simulink library "NeuroMuscularLibrary"  (R2019a)
settings: Solver=ode45  StartTime=0.0  StopTime=10.0  RelTol=1e-3  EnableMultiTasking=on
undefined symbols (not defined in the file): a2loptHAB, a2loptHAD, a2loptHAMsw, a2loptRFsw, ankle_height, aRefHAB, aRefHAD, aRefHAMsw, aRefRFsw, c, c_jointstop, deltaLegAngleThr, DeltaThRef, eref, Fmax, FmaxGLU, footBallToAnkleDist, footBallToCGDist, footBallToCGDist_y, footBallToHeelDist, footCenterlineToBall, footCenterlineToHeel, footInertia, footLength, footMass, FT, FT_GLU, GainDphiHATGLUst, GainDphiHATHABst, GainDphiHATHADst, GainDphiHATHFLst, GainFGASst, GainFGLUst, GainFHABst, GainFHAMst, GainFSOLst, GainFSOLTAst, GainFVASst, GainLBFSHst, GainLBFSHVASst, GainLGLUsw, GainLHABsw, GainLHADsw, GainLHAMGLUsw, GainLHAMsw, GainLRFHFLsw, GainLTAst, GainLTAsw, GainLVASsw, GainPhiHATGLUst, GainPhiHATHABst, GainPhiHATHADst, GainPhiHATHFLst, GainSGLUcHFLst, GainSGLUHAMst, GainSHABcHABst, GainSHADcHADst, GainSHAMBFSHsw, GainSHAMcHFLst, GainSHAMGASsw ... (+175)
libraries: sm_lib x54, $bdroot x45, nesl_utility x39, simulink x24, simulink_extras x6, vrlib x5, dspsigops x4
(part 1 of 5)
settings Model: Creator=nitisht  LastModifiedBy=Jesper
settings DataIOCC: LimitDataPoints=on  SaveFormat=Array  ReturnWorkspaceOutputs=off
settings OptimizationCC: LifeSpan=inf
settings DebuggingCC: UnderspecifiedInitializationDetection=Classic  MergeDetectMultiDrivingBlocksExec=none  SolverPrmCheckMsg=warning  StateNameClashWarn=warning  SFUnexpectedBacktrackingDiag=warning  SFNoUnconditionalDefaultTransitionDiag=warning  SFExecutionAtInitializationDiag=none  ArithmeticOperatorsInVariantConditions=warning
settings HardwareCC: ProdBitPerLong=64  ProdLargestAtomicFloat=None  ProdIntDivRoundTo=Undefined  ProdEndianess=Unspecified  ProdHWDeviceType=Intel->x86-64
settings ModelReferenceCC: PropagateSignalLabelsOutOfModel=off
settings SFSimCC: SimUseLocalCustomCode=off
settings RTWCC: RTWUseLocalCustomCode=off  RTWCompilerOptimization=on
settings CodeAppCC: StateflowObjectComments=on
settings GRTTargetCC: TargetLangStandard=C89/C90 (ANSI)
settings ConfigComp: CovMetricSettings=dw  CovHtmlReporting=on  CovSaveCumulativeToWorkspaceVar=on  CovSaveSingleToWorkspaceVar=on  CovExternalEMLEnable=off  CovSFcnEnable=off

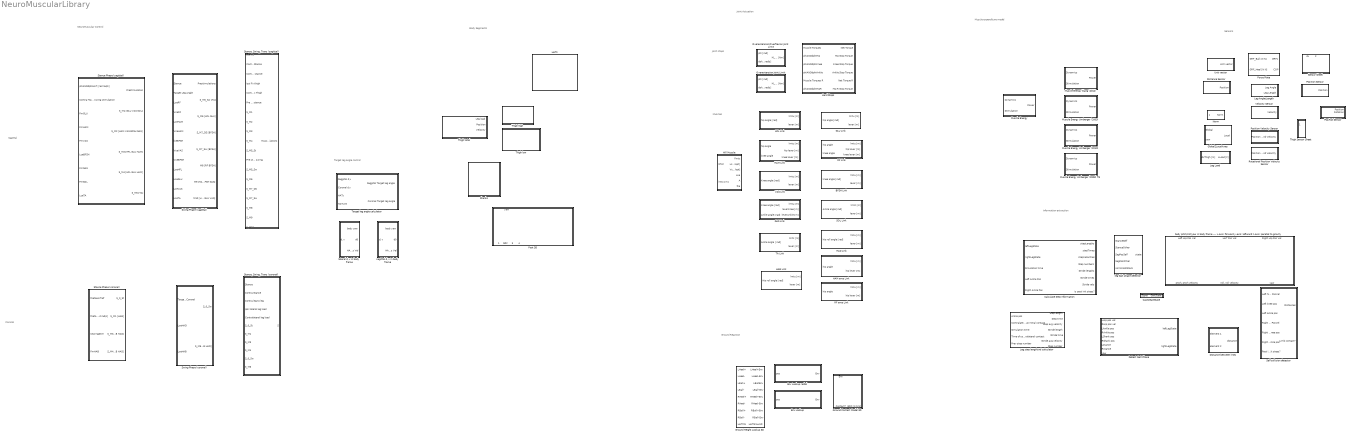
== system NeuroMuscularLibrary ==
  note: Body Segments
  note: Joint Actuation
  note: Sensors
  note: Ground Reaction
  note: NeuroMuscular Control
  note: Sagittal
  note: Coronal
  note: Muscle expenditure
      | model
  note: Joint stops
  note: Muscles
  note: Information extraction
  note: Target leg angle control
  BFSH Link : Subsystem
  Calculate Step information : Subsystem  mask{initiationSteps=innerOptSettings.initiationSteps}
      mask prompts: initiationSteps "Number of initiation steps"
  Cast2GaitState : Subsystem
  Detect Gait Phase : Subsystem
  Distance Sensor : Subsystem
  Distance between lines : Subsystem
  Env Lookup : Subsystem
  Env Lookup radial : Subsystem
  Foot 3D : Subsystem  mask{footMass=footMass, footInertia=footInertia, footSide=Left foot}
      mask prompts: footMass "Foot mass in kg"; footInertia "Foot inertia in kg*m^2"; footSide "Side"
      mask TypeOptions footSide: Left foot | Right foot
  Force Plate : Subsystem  TreatAsAtomicUnit=on
  GAS Link : Subsystem
  GLU Link : Subsystem
  Global2LocalAxes : Subsystem
  Ground Contact Model 3D : Subsystem
  Ground Height Lookup 3D : Subsystem
  HAB Link : Subsystem
  HAD Link : Subsystem
  HAM Link : Subsystem
  HAM amp Link : Subsystem
  HATs : Subsystem
  HFL Link : Subsystem
  Hard Stops : Subsystem
  Hill Muscle : Subsystem  mask(Hill Type Muscle){Fmax=Fmax, lopt=lopt, vmax=vmax, lslack=lslack}
      mask prompts: Fmax "Max Isometric Force [N]"; lopt "Optimal Length [m]"; vmax "Max Contraction Velocity [m/s]"; lslack "Slack Length [m]"
      mask help:
      | Hill Type Muscle Model. This dialog allows you to specify several muscle-specific parameters. The block also requires several parameters to be defined globally in the matlab workspace:
      |
      | Excitation-contraction coupling parameters:
      | preA: preactivation
      | tau:  delay time constant [s]
      |
      | Contractile element (CE) force-length relationship:
      | w: width [lopt]
      | c: remaining force at +/- width
      |
      | CE force-velocity parameters:
      | N: eccentric force enhancement [Fmax]
      | K: shape factor
      |
      | Series elastic element (SE) force-length relationship
      | eref: tendon reference strain [lslack]
  Leg Angle/Length : Subsystem
  Leg Load : Subsystem
  Leg step length/vel calculator : Subsystem
  Muscle Energy : Subsystem  mask{lopt=loptGLU, FT=FT_GLU, Fmax=FmaxGLU, vmax=vmaxGLU}
      mask prompts: lopt "Optimum Length:"; FT "Percent Fast Twitch"; Fmax "Max Iso Force"; vmax "Max Contraction Velocity in m/s"
  Muscle Energy Umberger (2003) : Subsystem  mask{lopt=lopt, FT=FT, Fmax=Fmax, vmax=vmax}
      mask prompts: lopt "Optimum Length:"; FT "Percent Fast Twitch"; Fmax "Max Iso Force"; vmax "Max Contraction Velocity in m/s"
  Muscle Energy Umberger (2003) TG : Subsystem  mask{lopt=loptGLU, FT=FT_GLU, Fmax=FmaxGLU}
      mask prompts: lopt "Optimum Length:"; FT "Percent Fast Twitch"; Fmax "Max Iso Force"
  Muscle Energy Umberger (2010) : Subsystem  mask{lopt=lopt, FT=FT, Fmax=Fmax, vmax=vmax}
      mask prompts: lopt "Optimum Length:"; FT "Percent Fast Twitch"; Fmax "Max Iso Force"; vmax "Max Contraction Velocity in m/s"
  Muscle Energy Wang (2012) : Subsystem  mask{lopt=lopt, FT=FT, Fmax=Fmax}
      mask prompts: lopt "Optimum Length:"; FT "Percent Fast Twitch"; Fmax "Max Iso Force"
  Norm : Subsystem
  Overextension Joint Limit : Subsystem  mask{phiUpLimit=phiKneeUpLimit, ext=1}
      mask prompts: phiUpLimit "Upper Limit [rad]"; ext "Extension values are positive or negative?"
      mask help:
      | This block implements a hard joint limit that will prevent the joint from extending past the specified upper limit.
      |
      | Used for the knee and hip joints.
  Overextension/Overflexion Joint Limit : Subsystem  mask(Overextension/Overflexion Joint Limit){phiUpLimit=0, phiLowLimit=0}
      mask prompts: phiUpLimit "Upper Limit [rad]"; phiLowLimit "Lower Limit [rad]"
      mask help:
      | This block implents a hard joint limit that will prevent the joint from overextending past the specified upper limit and overflexing below the lower limit.
      |
      | Used for the Ankle Joint.
  Pos/Rot Sensor : Subsystem
  Position Sensor : Subsystem
  Position Velocity Sensor : Subsystem
  RF Link : Subsystem
  RF amp Link : Subsystem
  Rotational Position Velocity Sensor : Subsystem
  SOL Link : Subsystem
  Self collision detector : Subsystem  mask{maxDist=innerOptSettings.minLimbDistance}
      mask prompts: maxDist "Minimal distance limbs (m)"
  Sensor Sheet : Subsystem
  Shanks : Subsystem
  Stance Phase (coronal) : Subsystem  TreatAsAtomicUnit=on  mask{PreStimHABst=PreStimHABst, PreStimHADst=PreStimHADst, GainFHABst=GainFHABst, GainPhiHATHABst=GainPhiHATHABst, GainDphiHATHABst=GainDphiHATHABst, GainPhiHATHADst=GainPhiHATHADst, GainDphiHATHADst=GainDphiHATHADst, GainSHABcHABst=GainSHABcHABst, GainSHADcHADst=GainSHADcHADst}
      mask DialogControl Container3 Prompt: Pre-stimulations
      mask DialogControl Container4 Prompt: M1: realize compliant leg
      mask DialogControl Container5 Prompt: M3: balance trunk
      mask DialogControl Container6 Prompt: M4: compensate swing leg
  Stance Phase (sagittal) : Subsystem  TreatAsAtomicUnit=on  mask{PreStimHFLst=PreStimHFLst, PreStimGLUst=PreStimGLUst, PreStimHAMst=PreStimHAMst, PreStimRFst=PreStimRFst, PreStimVASst=PreStimVASst, PreStimBFSHst=PreStimBFSHst, PreStimGASst=PreStimGASst, PreStimSOLst=PreStimSOLst, PreStimTAst=PreStimTAst, GainFGLUst=GainFGLUst, GainFVASst=GainFVASst, GainFSOLst=GainFSOLst, GainFHAMst=GainFHAMst, LceOffsetBFSHVASst=LceOffsetBFSHVASst, GainLBFSHVASst=GainLBFSHVASst, LceOffsetBFSHst=LceOffsetBFSHst, GainLBFSHst=GainLBFSHst, GainFGASst=GainFGASst, phiHATref=phiHATref, GainPhiHATHFLst=GainPhiHATHFLst, GainDphiHATHFLst=GainDphiHATHFLst, GainPhiHATGLUst=GainPhiHATGLUst, GainDphiHATGLUst=GainDphiHATGLUst, GainSGLUHAMst=GainSGLUHAMst, GainSGLUcHFLst=GainSGLUcHFLst, GainSHAMcHFLst=GainSHAMcHFLst, GainSHFLcGLUst=GainSHFLcGLUst, GainSRFcGLUst=GainSRFcGLUst, LceOffsetTAst=LceOffsetTAst, GainLTAst=GainLTAst, GainFSOLTAst=GainFSOLTAst}
      mask DialogControl Container3 Prompt: Pre-stimulations
      mask DialogControl Container4 Prompt: M1: realize compliant leg
      mask DialogControl Container5 Prompt: M2: prevent knee overextension
      mask DialogControl Container6 Prompt: M3: balance trunk
      mask DialogControl Container7 Prompt: M4: compensate swing leg
      mask DialogControl Container8 Prompt: M5: flex ankle
  "Stance, Swing, Trans (coronal)" : Subsystem  TreatAsAtomicUnit=on  mask{transSupst_C=transSupst_C, transsw_C=transsw_C}
  "Stance, Swing, Trans (sagittal)" : Subsystem  mask{transSupst=transSupst, transsw=transsw}
  Swing Phase (coronal) : Subsystem  TreatAsAtomicUnit=on  mask{PreStimHABsw=PreStimHABsw, PreStimHADsw=PreStimHADsw, GainLHABsw=GainLHABsw, GainLHADsw=GainLHADsw}
      mask DialogControl Container2 Prompt: Parameters
      mask DialogControl Container4 Prompt: Pre-stimulations
      mask DialogControl Container5 Prompt: M6: swing hip
  Swing Phase (sagittal) : Subsystem  TreatAsAtomicUnit=on  mask{PreStimHFLsw=PreStimHFLsw, PreStimGLUsw=PreStimGLUsw, PreStimHAMsw=PreStimHAMsw, PreStimRFsw=PreStimRFsw, PreStimVASsw=PreStimVASsw, PreStimBFSHsw=PreStimBFSHsw, PreStimGASsw=PreStimGASsw, PreStimSOLsw=PreStimSOLsw, PreStimTAsw=PreStimTAsw, GainLTAsw=GainLTAsw, LceOffsetTAsw=LceOffsetTAsw, GainLRFHFLsw=GainLRFHFLsw, GainVRFHFLsw=GainVRFHFLsw, GainLHAMGLUsw=GainLHAMGLUsw, GainVHAMGLUsw=GainVHAMGLUsw, GainVRFBFSHsw=GainVRFBFSHsw, GainVVASRFsw=GainVVASRFsw, GainVBFSHsw=GainVBFSHsw, GainLHAMsw=GainLHAMsw, GainSHAMBFSHsw=GainSHAMBFSHsw, GainSHAMGASsw=GainSHAMGASsw, SHAMthresholdsw=SHAMthresholdsw, GainLHFLsw=GainLGLUsw, GainLGLUsw=GainLGLUsw, LceOffsetVASsw=LceOffsetVASsw, GainLVASsw=GainLVASsw, legLengthClr=legLengthClr, deltaLegAngleThr=deltaLegAngleThr}
      mask DialogControl Container4 Prompt: Pre-stimulations
      mask DialogControl Container6 Prompt: M5: swing Ctrl (ankle)
      mask DialogControl Container5 Prompt: M6: swing Ctrl (hip)
      mask DialogControl Container7 Prompt: M7: swing Ctrl (knee_i)
      mask DialogControl Container8 Prompt: swing Ctrl (knee_ii)
      mask DialogControl Container9 Prompt: swing Ctrl (knee_iii)
      mask DialogControl Container10 Prompt: swing Ctrl (stance preparation)
      mask DialogControl Container12 Prompt: Foot placement
  TA Link : Subsystem
  Target leg angle calculator : Subsystem  mask{simbiconLegAngle0=LsimbiconLegAngle0, simbiconGainD=LsimbiconGainD, simbiconGainV=LsimbiconGainV, simbiconLegAngle0_C=LsimbiconLegAngle0_C, simbiconGainD_C=LsimbiconGainD_C, simbiconGainV_C=LsimbiconGainV_C, headingGain=0, headingIntGain=0}
      mask DialogControl Container3 Prompt: Saggital foot placement
      mask DialogControl Container4 Prompt: Coronal foot placement
  Thigh Sensor Sheet : Subsystem
  Thigh high : Subsystem  mask{thighLength=0, thighMass=0, thighInertiaHigh=0, thighKneeToCG=0}
      mask prompts: thighLength "Thigh length (in m)"; thighMass "Thigh mass (in kg)"; thighInertiaHigh "Upper thigh inertia (in kg m^2)"; thighKneeToCG "Distance knee to CG of thigh (in m)"
  Thigh low : Subsystem  mask{thighLength=0, thighMass=0, thighInertiaLow=0, thighKneeToCG=0}
      mask prompts: thighLength "Thigh length (in m)"; thighMass "Thigh mass (in kg)"; thighInertiaLow "Lower thigh inertia (in kg m^2)"; thighKneeToCG "Distance knee to CG of thigh (in m)"
  Thigh total : Subsystem
  Unit vector : Subsystem
  VAS Link : Subsystem
  Velocity Sensor : Subsystem
  body pitch/roll/yaw in body frame --- x-axis: forward y-axis: leftward z-axis: parallel to gravity : Subsystem
  "lateral d, v in body frame" : Subsystem
  leg Gait phase detector : Subsystem
  "sagittal d, v in body frame" : Subsystem

== system NeuroMuscularLibrary/BFSH Link ==
  note: BFSH Attachment
  knee angle [rad] : Inport
  Constant : Constant  Value=lslackBFSH+loptBFSH
  Constant1 : Constant  Value=rBFSH
  Constant2 : Constant  Value=phirefBFSH
  Gain2 : Gain  Gain=rhoBFSH
  Product : Product  RndMeth=Zero
  Sum2 : Sum  Inputs=|-+
  Sum5 : Sum  Inputs=|++
  lmtu [m] : Outport  VectorParamsAs1DForOutWhenUnconnected=on
  lever [m] : Outport  Port=2  VectorParamsAs1DForOutWhenUnconnected=on
  wires:
  Constant1/1 -> Product/2, lever [m]/1
  Constant/1 -> Sum5/1
  Constant2/1 -> Sum2/2
  Sum5/1 -> lmtu [m]/1
  Gain2/1 -> Sum5/2
  Product/1 -> Gain2/1
  knee angle [rad]/1 -> Sum2/1
  Sum2/1 -> Product/1

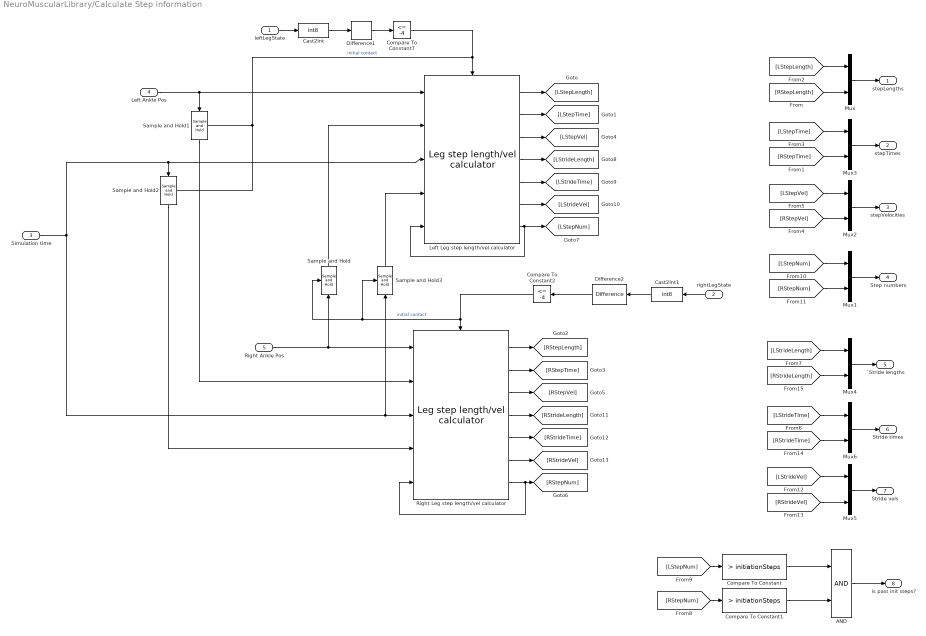
== system NeuroMuscularLibrary/Calculate Step information ==
  leftLegState : Inport
  rightLegState : Inport  Port=2
  Simulation time : Inport  Port=3
  Left Ankle Pos : Inport  Port=4
  "Right Ankle Pos " : Inport  Port=5
  AND : Logic  AllPortsSameDT=off  OutDataTypeStr=boolean
  Cast2Int : DataTypeConversion  OutDataTypeStr=int8
  Cast2Int1 : DataTypeConversion  OutDataTypeStr=int8
  Compare To Constant : simulink/Logic and Bit Operations/Compare To Constant  relop=>  const=initiationSteps  OutDataTypeStr=boolean  ZeroCross=off
  Compare To Constant1 : simulink/Logic and Bit Operations/Compare To Constant  relop=>  const=initiationSteps  OutDataTypeStr=boolean  ZeroCross=off
  Compare To Constant2 : simulink/Logic and Bit Operations/Compare To Constant  relop=<=  const=-4  OutDataTypeStr=boolean
  Compare To Constant7 : simulink/Logic and Bit Operations/Compare To Constant  relop=<=  const=-4  OutDataTypeStr=boolean
  Difference1 : simulink/Discrete/Difference  ICPrevInput=0.0  OutMin=[]  OutMax=[]  OutDataType=fixdt(1, 16)  OutScaling=2^-10  DoSatur=off
  Difference2 : simulink/Discrete/Difference  ICPrevInput=0.0  OutMin=[]  OutMax=[]  OutDataType=fixdt(1, 16)  OutScaling=2^-10  DoSatur=off
  Left Leg step length/vel calculator : $bdroot/Leg step length//vel calculator  SystemSampleTime=-1  Latency=0  AutoFrameSizeCalculation=off
  Mux{,1..6} (7 alike) : Mux  Inputs=2
  Right Leg step length/vel calculator : $bdroot/Leg step length//vel calculator  SystemSampleTime=-1  Latency=0  AutoFrameSizeCalculation=off
  Sample and Hold{,1..3} (4 alike) : dspsigops/Sample and Hold  trig=Rising edge  initCond=0  latchinput=off
  stepLengths : Outport  VectorParamsAs1DForOutWhenUnconnected=on
  stepTimes : Outport  Port=2  VectorParamsAs1DForOutWhenUnconnected=on
  stepVelocities : Outport  Port=3  VectorParamsAs1DForOutWhenUnconnected=on
  Step numbers : Outport  Port=4  VectorParamsAs1DForOutWhenUnconnected=on
  `Stride lengths : Outport  Port=5  VectorParamsAs1DForOutWhenUnconnected=on
  Stride times : Outport  Port=6  VectorParamsAs1DForOutWhenUnconnected=on
  Stride vels : Outport  Port=7  VectorParamsAs1DForOutWhenUnconnected=on
  is past init steps? : Outport  Port=8  VectorParamsAs1DForOutWhenUnconnected=on
  wires:
  Right Leg step length/vel calculator/1 -> [RStepLength]
  Left Leg step length/vel calculator/1 -> [LStepLength]
  Simulation time/1 -> Right Leg step length/vel calculator/3, Sample and Hold3/1, Left Leg step length/vel calculator/3, Sample and Hold2/1
  Compare To Constant7/1 -> Sample and Hold1/Trigger, Sample and Hold2/Trigger, Left Leg step length/vel calculator/Enable  "initial contact"
  Right Leg step length/vel calculator/3 -> [RStepVel]
  Compare To Constant2/1 -> Sample and Hold3/Trigger, Sample and Hold/Trigger, Right Leg step length/vel calculator/Enable  "initial contact"
  Mux2/1 -> stepVelocities/1
  Left Leg step length/vel calculator/3 -> [LStepVel]
  Right Leg step length/vel calculator/2 -> [RStepTime]
  Difference2/1 -> Compare To Constant2/1
  Mux/1 -> stepLengths/1
  Left Leg step length/vel calculator/2 -> [LStepTime]
  Mux3/1 -> stepTimes/1
  leftLegState/1 -> Cast2Int/1
  Compare To Constant1/1 -> AND/2
  Compare To Constant/1 -> AND/1
  AND/1 -> is past init steps?/1
  Left Ankle Pos/1 -> Left Leg step length/vel calculator/1, Sample and Hold1/1
  "Right Ankle Pos "/1 -> Right Leg step length/vel calculator/1, Sample and Hold/1
  Difference1/1 -> Compare To Constant7/1
  rightLegState/1 -> Cast2Int1/1
  [RStepLength] -> Mux/2
  [LStepLength] -> Mux/1
  [LStepTime] -> Mux3/1
  [RStepTime] -> Mux3/2
  [RStepVel] -> Mux2/2
  [LStepVel] -> Mux2/1
  Left Leg step length/vel calculator/7 -> [LStepNum], Left Leg step length/vel calculator/5
  Right Leg step length/vel calculator/7 -> Right Leg step length/vel calculator/5, [RStepNum]
  [LStepNum] -> Compare To Constant/1
  [RStepNum] -> Compare To Constant1/1
  Mux1/1 -> Step numbers/1
  [LStepNum] -> Mux1/1
  [RStepNum] -> Mux1/2
  Left Leg step length/vel calculator/4 -> [LStrideLength]
  Left Leg step length/vel calculator/5 -> [LStrideTime]
  Left Leg step length/vel calculator/6 -> [LStrideVel]
  Right Leg step length/vel calculator/4 -> [RStrideLength]
  Right Leg step length/vel calculator/5 -> [RStrideTime]
  Right Leg step length/vel calculator/6 -> [RStrideVel]
  Sample and Hold/1 -> Left Leg step length/vel calculator/2
  Sample and Hold1/1 -> Right Leg step length/vel calculator/2
  Sample and Hold3/1 -> Left Leg step length/vel calculator/4
  Sample and Hold2/1 -> Right Leg step length/vel calculator/4
  [LStrideVel] -> Mux5/1
  [RStrideLength] -> Mux4/2
  [LStrideTime] -> Mux6/1
  [RStrideTime] -> Mux6/2
  Mux4/1 -> `Stride lengths/1
  [LStrideLength] -> Mux4/1
  Mux6/1 -> Stride times/1
  Mux5/1 -> Stride vels/1
  [RStrideVel] -> Mux5/2
  Cast2Int/1 -> Difference1/1
  Cast2Int1/1 -> Difference2/1

== system NeuroMuscularLibrary/Cast2GaitState ==
  Signal : Inport
  Cast2GaitState : DataTypeConversion  OutDataTypeStr=Enum: GaitState
  Cast2Int : DataTypeConversion  OutDataTypeStr=int8
  GaitState : Outport  OutDataTypeStr=Enum: GaitState  VectorParamsAs1DForOutWhenUnconnected=on
  wires:
  Cast2Int/1 -> Cast2GaitState/1
  Cast2GaitState/1 -> GaitState/1
  Signal/1 -> Cast2Int/1

== system NeuroMuscularLibrary/Detect Gait Phase ==
  LHip pos vel : Inport
  RHip pos vel : Inport  Port=2
  LAnkle pos : Inport  Port=3
  RAnkle pos : Inport  Port=4
  LShank pos : Inport  Port=5
  RShank pos : Inport  Port=6
  Lstance : Inport  Port=7
  Rstance : Inport  Port=8
  yaw : Inport  Port=9
  Add : Sum  Inputs=+-
  Add1 : Sum  Inputs=-+
  Add2 : Sum  Inputs=+-
  Add3 : Sum  Inputs=+-
  Add4 : Sum
  Left leg Gait phase detector : $bdroot/leg Gait phase detector  SystemSampleTime=-1  Latency=0  AutoFrameSizeCalculation=off
  Multiply : Gain  Gain=1/2
  Mux : Mux  Inputs=2
  Mux1 : Mux  Inputs=2
  Norm : Fcn  Expr=sqrt( u(1)^2 + u(2)^2 + u(3)^2 )
  Norm1 : Fcn  Expr=sqrt( u(1)^2 + u(2)^2 + u(3)^2 )
  Right leg Gait phase detector : $bdroot/leg Gait phase detector  SystemSampleTime=-1  Latency=0  AutoFrameSizeCalculation=off
  Selector : Selector  InputPortWidth=3  IndexOptions=Index vector (dialog)  Indices=[1 2]  OutputSizes=1
  Selector1 : Selector  InputPortWidth=3  IndexOptions=Index vector (dialog)  Indices=[1 2]  OutputSizes=1
  Selector4 : Selector  InputPortWidth=6  IndexOptions=Index vector (dialog)  Indices=[1 2 3]  OutputSizes=1
  body frame in transverse plane (xz-plane) : Fcn  Expr=u(1)*cos(u(3)) + u(2)*sin(u(3))
  body frame in transverse plane (xz-plane)1 : Fcn  Expr=u(2)*cos(u(1)) + u(3)*sin(u(1))
  leftLegState : Outport  VectorParamsAs1DForOutWhenUnconnected=on
  rightLegState : Outport  Port=2  VectorParamsAs1DForOutWhenUnconnected=on
  wires:
  LAnkle pos/1 -> Add2/1, Add/1
  RAnkle pos/1 -> Add1/2, Add3/1
  Add/1 -> Selector/1
  Selector/1 -> Mux/1  "(x,y)"
  Add1/1 -> Selector1/1
  Selector1/1 -> Mux1/2  "x,y)"
  LShank pos/1 -> Add2/2
  RShank pos/1 -> Add3/2
  Add3/1 -> Norm1/1
  Add2/1 -> Norm/1
  Add4/1 -> Selector4/1
  Multiply/1 -> Add/2, Add1/1
  LHip pos vel/1 -> Add4/1
  RHip pos vel/1 -> Add4/2
  Selector4/1 -> Multiply/1
  Mux/1 -> body frame in transverse plane (xz-plane)/1
  Mux1/1 -> body frame in transverse plane (xz-plane)1/1
  yaw/1 -> Mux/2, Mux1/1
  body frame in transverse plane (xz-plane)/1 -> [LsagPos]
  body frame in transverse plane (xz-plane)1/1 -> [RsagPos]
  Lstance/1 -> Right leg Gait phase detector/2, Left leg Gait phase detector/1
  Norm1/1 -> [RnormFootShank]
  Norm/1 -> [LnormFootShank]
  [LsagPos] -> Left leg Gait phase detector/3
  [LsagPos] -> Right leg Gait phase detector/4
  [RsagPos] -> Right leg Gait phase detector/3
  [RsagPos] -> Left leg Gait phase detector/4
  [LnormFootShank] -> Left leg Gait phase detector/5
  [RnormFootShank] -> Right leg Gait phase detector/5
  Rstance/1 -> Left leg Gait phase detector/2, Right leg Gait phase detector/1
  Right leg Gait phase detector/1 -> rightLegState/1
  Left leg Gait phase detector/1 -> leftLegState/1

== system NeuroMuscularLibrary/Distance Sensor ==
  PS-Simulink Converter : nesl_utility/PS-Simulink Converter  PhysicalDomain=network_engine_domain  SubClassName=ps_output  LeftPortType=input  RightPortType=output  PseudoPeriodic=off  Frequencies=[]  Unit=m  AffineConversion=off
  Position Sensor : sm_lib/Frames and Transforms/Transform Sensor  MeasurementFrame=World  SenseAngle=off  SenseAxis=off  SenseAngle1=off  SenseAngle2=off  SenseAngle3=off  SenseQ=off  SenseR=off  SenseOmegaX=off  SenseOmegaY=off  SenseOmegaZ=off  SenseOmega1=off  SenseOmega2=off  SenseOmega3=off  SenseQDot=off  SenseRDot=off  SenseAlphaX=off  SenseAlphaY=off  SenseAlphaZ=off  SenseAlpha1=off  SenseAlpha2=off  SenseAlpha3=off  SenseQDDot=off  SenseRDDot=off  SenseX=off  SenseY=off  SenseZ=off  SenseRad=off  SenseAzim=off  SenseDist=on  SenseInc=off  SenseXDot=off  SenseYDot=off  SenseZDot=off  SenseRadDot=off  SenseAzimDot=off  SenseDistDot=off  SenseIncDot=off  SenseXDDot=off  SenseYDDot=off  SenseZDDot=off  SenseRadDDot=off  SenseAzimDDot=off  SenseDistDDot=off  SenseIncDDot=off
  Base : PMIOPort  Side=Left
  Frame : PMIOPort  Port=2  Side=Left
  Position : Outport  VectorParamsAs1DForOutWhenUnconnected=on
  wires:
  PS-Simulink Converter/1 -> Position/1
  connections:
  Base/RConn1 -- Position Sensor/LConn1
  Position Sensor/RConn1 -- Frame/RConn1
  Position Sensor/RConn2 -- PS-Simulink Converter/LConn1

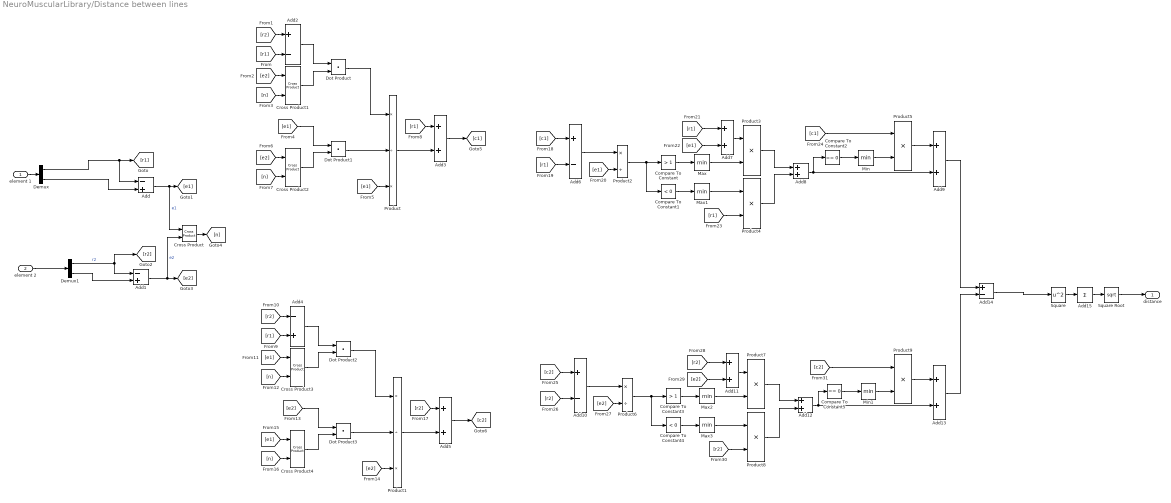
== system NeuroMuscularLibrary/Distance between lines ==
  element 1 : Inport
  element 2 : Inport  Port=2
  Add : Sum  Inputs=-+
  Add1 : Sum  Inputs=-+
  Add{2,6,10,14} (4 alike) : Sum  Inputs=+-
  Add{3,5,7..9,11..13} (8 alike) : Sum
  Add15 : Sum  Inputs=+  CollapseMode=Specified dimension
  Add4 : Sum  Inputs=-+
  Compare To Constant : simulink/Logic and Bit Operations/Compare To Constant  relop=>  const=1  OutDataTypeStr=uint8
  Compare To Constant1 : simulink/Logic and Bit Operations/Compare To Constant  relop=<  const=0  OutDataTypeStr=uint8
  Compare To Constant2 : simulink/Logic and Bit Operations/Compare To Constant  relop===  const=0  OutDataTypeStr=uint8
  Compare To Constant3 : simulink/Logic and Bit Operations/Compare To Constant  relop=>  const=1  OutDataTypeStr=uint8
  Compare To Constant4 : simulink/Logic and Bit Operations/Compare To Constant  relop=<  const=0  OutDataTypeStr=uint8
  Compare To Constant5 : simulink/Logic and Bit Operations/Compare To Constant  relop===  const=0  OutDataTypeStr=uint8
  Cross Product{,1..4} (5 alike) : vrlib/Utilities/Cross Product
  Demux : Demux  Outputs=2
  Demux1 : Demux  Outputs=2
  Dot Product{,1..3} (4 alike) : DotProduct  InputSameDT=on  OutDataTypeStr=Inherit: Inherit via internal rule
  Max{,1..3} (4 alike) : MinMax
  Min : MinMax
  Min1 : MinMax
  Product : Product  Inputs=*/*
  Product1 : Product  Inputs=*/*
  Product2 : Product  Inputs=*/
  Product{3..5,7..9} (6 alike) : Product
  Product6 : Product  Inputs=*/
  Square : Math  Operator=square  SaturateOnIntegerOverflow=on
  Square Root : Sqrt  SaturateOnIntegerOverflow=on
  distance : Outport  VectorParamsAs1DForOutWhenUnconnected=on
  wires:
  Demux/2 -> Add/2
  Demux1/2 -> Add1/2
  Demux1/1 -> [r2], Add1/1  "r2"
  Add/1 -> Cross Product/1, [e1]  "e1"
  Add1/1 -> Cross Product/2, [e2]  "e2"
  Cross Product/1 -> [n]
  [r2] -> Add2/1
  [r1] -> Add2/2
  [e2] -> Cross Product1/1
  [n] -> Cross Product1/2
  Add2/1 -> Dot Product/1
  Cross Product1/1 -> Dot Product/2
  Cross Product2/1 -> Dot Product1/2
  [e1] -> Dot Product1/1
  [n] -> Cross Product2/2
  [e2] -> Cross Product2/1
  Dot Product/1 -> Product/1
  Dot Product1/1 -> Product/2
  [e1] -> Product/3
  [r1] -> Add3/1
  Product/1 -> Add3/2
  Add3/1 -> [c1]
  Add5/1 -> [c2]
  Product1/1 -> Add5/2
  [r2] -> Add5/1
  [e2] -> Product1/3
  Dot Product3/1 -> Product1/2
  Dot Product2/1 -> Product1/1
  [e1] -> Cross Product4/1
  [n] -> Cross Product4/2
  [e2] -> Dot Product3/1
  Cross Product4/1 -> Dot Product3/2
  Cross Product3/1 -> Dot Product2/2
  Add4/1 -> Dot Product2/1
  [n] -> Cross Product3/2
  [e1] -> Cross Product3/1
  [r1] -> Add4/2
  [r2] -> Add4/1
  [r1] -> Add6/2
  [c1] -> Add6/1
  Add6/1 -> Product2/1
  [e1] -> Product2/2
  Product2/1 -> Compare To Constant1/1, Compare To Constant/1
  Compare To Constant/1 -> Max/1
  Compare To Constant1/1 -> Max1/1
  Max/1 -> Product3/2
  Add7/1 -> Product3/1
  [e1] -> Add7/2
  [r1] -> Add7/1
  Max1/1 -> Product4/1
  [r1] -> Product4/2
  Product4/1 -> Add8/2
  Product3/1 -> Add8/1
  [c1] -> Product5/1
  Add8/1 -> Add9/2, Compare To Constant2/1
  Compare To Constant2/1 -> Min/1
  Product5/1 -> Add9/1
  Add9/1 -> Add14/1
  Add12/1 -> Add13/2, Compare To Constant5/1
  Product9/1 -> Add13/1
  [r2] -> Add10/2
  Product8/1 -> Add12/2
  Compare To Constant5/1 -> Min1/1
  [c2] -> Add10/1
  Max2/1 -> Product7/2
  Add13/1 -> Add14/2
  Product7/1 -> Add12/1
  [e2] -> Add11/2
  Add11/1 -> Product7/1
  Compare To Constant3/1 -> Max2/1
  Add10/1 -> Product6/1
  [r2] -> Product8/2
  Product6/1 -> Compare To Constant4/1, Compare To Constant3/1
  Compare To Constant4/1 -> Max3/1
  [r2] -> Add11/1
  Max3/1 -> Product8/1
  [e2] -> Product6/2
  [c2] -> Product9/1
  Add14/1 -> Square/1
  Square Root/1 -> distance/1
  element 1/1 -> Demux/1
  Demux/1 -> Add/1, [r1]
  element 2/1 -> Demux1/1
  Add15/1 -> Square Root/1
  Square/1 -> Add15/1
  Min/1 -> Product5/2
  Min1/1 -> Product9/2

== system NeuroMuscularLibrary/Env Lookup ==
  note: environment lookup
  pos : Inport
  Constant : Constant  Value=0
  Gain : Gain  Gain=-1
  Ground Slope : Interpolation_n-D  NumberOfTableDimensions=1  Table=groundTheta  InterpMethod=Flat
      settings: InputPortMap=u0,u1
  Ground Z : Interpolation_n-D  NumberOfTableDimensions=1  Table=groundZ
      settings: InputPortMap=u0,u1
  Mux : Mux  Inputs=3
  Mux1 : Mux  Inputs=3
  Mux8 : Mux  Inputs=[1 3 3]
  Prelookup : PreLookup  BreakpointsData=groundX  BeginIndexSearchUsingPreviousIndexResult=on  ExtrapMethod=Linear  RndMeth=Simplest
  Selector1 : Selector  InputPortWidth=3  IndexOptions=Index vector (dialog)  Indices=[2]  OutputSizes=1
  Selector2 : Selector  InputPortWidth=3  IndexOptions=Index vector (dialog)  Indices=[1]  OutputSizes=1
  Trigonometric Function1 : Trigonometry
  Trigonometric Function2 : Trigonometry  Operator=cos
  Env : Outport  VectorParamsAs1DForOutWhenUnconnected=on
  wires:
  Constant/1 -> Mux1/2
  Mux1/1 -> Mux8/3  "Normal Vector"
  Selector1/1 -> Mux/2  "y"
  Mux/1 -> Mux8/2  "Reference Point"
  pos/1 -> Selector2/1, Selector1/1
  Prelookup/2 -> Ground Slope/2, Ground Z/2
  Trigonometric Function1/1 -> Gain/1
  Gain/1 -> Mux1/1  "Normal Vector x"
  Ground Slope/1 -> Trigonometric Function2/1, Trigonometric Function1/1
  Prelookup/1 -> Ground Slope/1, Ground Z/1
  Trigonometric Function2/1 -> Mux1/3  "Normal Vector z"
  Selector2/1 -> Prelookup/1, Mux/1  "x"
  Ground Z/1 -> Mux8/1, Mux/3  "Ground Height"
  Mux8/1 -> Env/1

== system NeuroMuscularLibrary/Env Lookup radial ==
  note: environment lookup
  pos : Inport
  Distance from world : Math  Operator=hypot  SaturateOnIntegerOverflow=on
  Gain1 : Gain  Gain=-1
  Ground Slope1 : Interpolation_n-D  NumberOfTableDimensions=1  Table=groundTheta  InterpMethod=Flat
      settings: InputPortMap=u0,u1
  Ground Z1 : Interpolation_n-D  NumberOfTableDimensions=1  Table=groundZ
      settings: InputPortMap=u0,u1
  Mux2 : Mux  Inputs=3
  Mux3 : Mux  Inputs=3
  Mux4 : Mux  Inputs=[1 3 3]
  Prelookup1 : PreLookup  BreakpointsData=groundX  BeginIndexSearchUsingPreviousIndexResult=on  ExtrapMethod=Linear  RndMeth=Simplest
  Product : Product  Inputs=/**
  Product1 : Product  Inputs=/**
  Selector3 : Selector  InputPortWidth=3  IndexOptions=Index vector (dialog)  Indices=[2]  OutputSizes=1
  Selector4 : Selector  InputPortWidth=3  IndexOptions=Index vector (dialog)  Indices=[1]  OutputSizes=1
  Trigonometric Function3 : Trigonometry
  Trigonometric Function4 : Trigonometry  Operator=cos
  Env : Outport  VectorParamsAs1DForOutWhenUnconnected=on
  wires:
  Mux3/1 -> Mux4/3  "Normal Vector"
  Ground Z1/1 -> Mux2/3, Mux4/1  "Ground Height"
  Mux4/1 -> Env/1
  Selector3/1 -> Mux2/2, Product1/2, Distance from world/2  "y"
  Trigonometric Function4/1 -> Mux3/3  "Normal Vector z"
  Prelookup1/1 -> Ground Z1/1, Ground Slope1/1
  Ground Slope1/1 -> Trigonometric Function4/1, Trigonometric Function3/1
  Mux2/1 -> Mux4/2  "Reference Point"
  pos/1 -> Selector4/1, Selector3/1
  Gain1/1 -> Product/3, Product1/3  "Normal Vector x/y"
  Prelookup1/2 -> Ground Z1/2, Ground Slope1/2
  Selector4/1 -> Mux2/1, Product/2, Distance from world/1  "x"
  Trigonometric Function3/1 -> Gain1/1
  Distance from world/1 -> Product1/1, Product/1, Prelookup1/1  "mag(x,y)"
  Product/1 -> Mux3/1  "Normal Vector x"
  Product1/1 -> Mux3/2  "Normal Vector y"

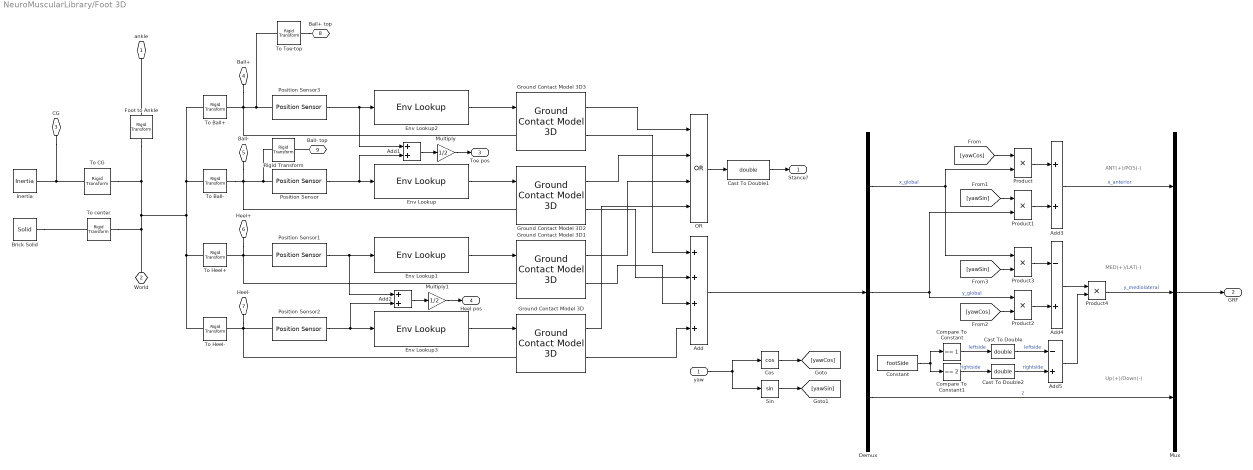
== system NeuroMuscularLibrary/Foot 3D ==
  note: ANT(+)/POS(-)
  note: MED(+)/LAT(-)
  note: Up(+)/Down(-)
  yaw : Inport
  Add : Sum  Inputs=++++
  Add1 : Sum
  Add2 : Sum
  Add3 : Sum
  Add4 : Sum  Inputs=-+
  Add5 : Sum  Inputs=-+
  Brick Solid : sm_lib/Body Elements/Solid  InertiaType=CalculateFromGeometry  Mass=0  MassUnits=kg  CenterOfMass=[0 0 0]  CenterOfMassUnits=m  MomentsOfInertia=[1 1 1]  MomentsOfInertiaUnits=kg*m^2  ProductsOfInertia=[0 0 0]  ProductsOfInertiaUnits=kg*m^2  BasedOnType=Mass  Density=0  DensityUnits=kg/m^3  DoExposeReferenceFrame=on  SerializedFrames=<Frames/>  GraphicType=FromGeometry  MarkerShape=Sphere  MarkerSize=10  GraphicVisPropType=SimpleVisualProperties  GraphicDiffuseColor=[0.5 0.5 0.5]  GraphicSpecularColor=[0.5 0.5 0.5 1.0]  GraphicAmbientColor=[0.15 0.15 0.15 1.0]  GraphicEmissiveColor=[0.0 0.0 0.0 1.0]  GraphicShininess=75  GraphicOpacity=1.0  GeometryShape=Brick  RectangleSize=[1 1]  RectangleSizeUnits=m  BrickDimensions=[footLength ankle_height footCenterlineToBall*2]  BrickDimensionUnits=m  CylinderRadius=1  CylinderRadiusUnits=m  CylinderLength=1  CylinderLengthUnits=m  SphereRadius=1  SphereRadiusUnits=m  EllipsoidRadii=[1 1 1]  EllipsoidRadiiUnits=m  ExtrusionCrossSection=[1 1; -1 1; -1 -1; 1 -1]  ExtrusionCrossSectionUnits=m  ExtrusionLength=1  ExtrusionLengthUnits=m  PolygonNumSides=3  PolygonOuterRadius=1  PolygonOuterRadiusUnits=m  ExtGeomFileType=STEP  ExtGeomFileUnits=m  RevolutionCrossSection=[1 1; 1 -1; 2 -1; 2 1]  RevolutionCrossSectionUnits=m  RevolutionExtent=Full  RevolutionAngle=180  RevolutionAngleUnits=deg
  Cast To Double : DataTypeConversion  OutDataTypeStr=double
  Cast To Double1 : DataTypeConversion  OutDataTypeStr=double
  Cast To Double2 : DataTypeConversion  OutDataTypeStr=double
  Compare To Constant : simulink/Logic and Bit Operations/Compare To Constant  relop===  const=1  OutDataTypeStr=uint8
  Compare To Constant1 : simulink/Logic and Bit Operations/Compare To Constant  relop===  const=2  OutDataTypeStr=uint8
  Constant : Constant  Value=footSide
  Cos : Trigonometry  Operator=cos
  Demux : Demux  Outputs=3
  Env Lookup{,1..3} (4 alike) : $bdroot/Env Lookup  SystemSampleTime=-1
  Foot to Ankle : sm_lib/Frames and Transforms/Rigid Transform  TranslationMethod=Cartesian  TranslationStandardOffset=0  TranslationLengthUnit=m  TranslationStandardAxis=+Z  TranslationCartesianOffset=[-footBallToAnkleDist ankle_height 0]  TranslationROffset=0  TranslationROffsetUnits=m  TranslationZOffset=0  TranslationZOffsetUnits=m  TranslationThetaOffset=0  TranslationThetaOffsetUnits=deg  RotationMethod=AlignedAxes  RotationAngleUnits=deg  RotationStandardAxis=+Z  RotationAngle=0.0  RotationArbitraryAxis=[0 0 1]  FollAlignAxisA=+Z  BaseAlignAxisA=+Z  FollAlignAxisB=+X  BaseAlignAxisB=+Y  RotationSequenceAxes=FollowerAxes  RotationSequence=XYX  RotationSequenceAngles=[0 0 0]  RotationSequenceAnglesUnits=deg  RotationMatrix=[1 0 0; 0 1 0; 0 0 1]
  Ground Contact Model 3D{,1..3} (4 alike) : $bdroot/Ground Contact Model 3D  SystemSampleTime=-1
  Inertia : sm_lib/Body Elements/Inertia  InertiaType=Custom  Mass=footMass  MassUnits=kg  CenterOfMass=[0 0 0]  CenterOfMassUnits=m  MomentsOfInertia=footInertia  MomentsOfInertiaUnits=kg*m^2  ProductsOfInertia=[0 0 0]  ProductsOfInertiaUnits=kg*m^2  GraphicType=None  MarkerShape=Inertia  MarkerSize=20  GraphicVisPropType=SimpleVisualProperties  GraphicDiffuseColor=[0.5 0.5 0.5]  GraphicSpecularColor=[0.5 0.5 0.5 1.0]  GraphicAmbientColor=[0.15 0.15 0.15 1.0]  GraphicEmissiveColor=[0.0 0.0 0.0 1.0]  GraphicShininess=75  GraphicOpacity=1.0
  Multiply : Gain  Gain=1/2
  Multiply1 : Gain  Gain=1/2
  Mux : Mux  Inputs=3
  OR : Logic  Operator=OR  Inputs=4  AllPortsSameDT=off  OutDataTypeStr=boolean
  Position Sensor{,1..3} (4 alike) : $bdroot/Position Sensor  SystemSampleTime=-1
  Product{,1..4} (5 alike) : Product
  Rigid Transform : sm_lib/Frames and Transforms/Rigid Transform  TranslationMethod=Cartesian  TranslationStandardOffset=0  TranslationLengthUnit=m  TranslationStandardAxis=+Z  TranslationCartesianOffset=[0 ankle_height 0]  TranslationROffset=0  TranslationROffsetUnits=m  TranslationZOffset=0  TranslationZOffsetUnits=m  TranslationThetaOffset=0  TranslationThetaOffsetUnits=deg  RotationMethod=None  RotationAngleUnits=deg  RotationStandardAxis=+Z  RotationAngle=0.0  RotationArbitraryAxis=[0 0 1]  FollAlignAxisA=+X  BaseAlignAxisA=+Y  FollAlignAxisB=+Y  BaseAlignAxisB=+Z  RotationSequenceAxes=FollowerAxes  RotationSequence=XYX  RotationSequenceAngles=[0 0 0]  RotationSequenceAnglesUnits=deg  RotationMatrix=[1 0 0; 0 1 0; 0 0 1]
  Sin : Trigonometry
  To Ball+ : sm_lib/Frames and Transforms/Rigid Transform  TranslationMethod=Cartesian  TranslationStandardOffset=0  TranslationLengthUnit=m  TranslationStandardAxis=+Z  TranslationCartesianOffset=[0 0 footCenterlineToBall]  TranslationROffset=0  TranslationROffsetUnits=m  TranslationZOffset=0  TranslationZOffsetUnits=m  TranslationThetaOffset=0  TranslationThetaOffsetUnits=deg  RotationMethod=None  RotationAngleUnits=deg  RotationStandardAxis=+Z  RotationAngle=0.0  RotationArbitraryAxis=[0 0 1]  FollAlignAxisA=+X  BaseAlignAxisA=+Y  FollAlignAxisB=+Y  BaseAlignAxisB=+Z  RotationSequenceAxes=FollowerAxes  RotationSequence=XYX  RotationSequenceAngles=[0 0 0]  RotationSequenceAnglesUnits=deg  RotationMatrix=[1 0 0; 0 1 0; 0 0 1]
  To Ball- : sm_lib/Frames and Transforms/Rigid Transform  TranslationMethod=Cartesian  TranslationStandardOffset=0  TranslationLengthUnit=m  TranslationStandardAxis=+Z  TranslationCartesianOffset=[0 0 -footCenterlineToBall]  TranslationROffset=0  TranslationROffsetUnits=m  TranslationZOffset=0  TranslationZOffsetUnits=m  TranslationThetaOffset=0  TranslationThetaOffsetUnits=deg  RotationMethod=None  RotationAngleUnits=deg  RotationStandardAxis=+Z  RotationAngle=0.0  RotationArbitraryAxis=[0 0 1]  FollAlignAxisA=+X  BaseAlignAxisA=+Y  FollAlignAxisB=+Y  BaseAlignAxisB=+Z  RotationSequenceAxes=FollowerAxes  RotationSequence=XYX  RotationSequenceAngles=[0 0 0]  RotationSequenceAnglesUnits=deg  RotationMatrix=[1 0 0; 0 1 0; 0 0 1]
  To CG : sm_lib/Frames and Transforms/Rigid Transform  TranslationMethod=Cartesian  TranslationStandardOffset=0  TranslationLengthUnit=m  TranslationStandardAxis=+Z  TranslationCartesianOffset=[-footBallToCGDist footBallToCGDist_y 0]  TranslationROffset=0  TranslationROffsetUnits=m  TranslationZOffset=0  TranslationZOffsetUnits=m  TranslationThetaOffset=0  TranslationThetaOffsetUnits=deg  RotationMethod=AlignedAxes  RotationAngleUnits=deg  RotationStandardAxis=+Z  RotationAngle=0.0  RotationArbitraryAxis=[0 0 1]  FollAlignAxisA=+Z  BaseAlignAxisA=+Y  FollAlignAxisB=+X  BaseAlignAxisB=+X  RotationSequenceAxes=FollowerAxes  RotationSequence=XYX  RotationSequenceAngles=[0 0 0]  RotationSequenceAnglesUnits=deg  RotationMatrix=[1 0 0; 0 1 0; 0 0 1]
  To Heel+ : sm_lib/Frames and Transforms/Rigid Transform  TranslationMethod=Cartesian  TranslationStandardOffset=0  TranslationLengthUnit=m  TranslationStandardAxis=+Z  TranslationCartesianOffset=[-footBallToHeelDist 0 footCenterlineToHeel]  TranslationROffset=0  TranslationROffsetUnits=m  TranslationZOffset=0  TranslationZOffsetUnits=m  TranslationThetaOffset=0  TranslationThetaOffsetUnits=deg  RotationMethod=None  RotationAngleUnits=deg  RotationStandardAxis=+Z  RotationAngle=0.0  RotationArbitraryAxis=[0 0 1]  FollAlignAxisA=+X  BaseAlignAxisA=+Y  FollAlignAxisB=+Y  BaseAlignAxisB=+Z  RotationSequenceAxes=FollowerAxes  RotationSequence=XYX  RotationSequenceAngles=[0 0 0]  RotationSequenceAnglesUnits=deg  RotationMatrix=[1 0 0; 0 1 0; 0 0 1]
  To Heel- : sm_lib/Frames and Transforms/Rigid Transform  TranslationMethod=Cartesian  TranslationStandardOffset=0  TranslationLengthUnit=m  TranslationStandardAxis=+Z  TranslationCartesianOffset=[-footBallToHeelDist 0 -footCenterlineToHeel]  TranslationROffset=0  TranslationROffsetUnits=m  TranslationZOffset=0  TranslationZOffsetUnits=m  TranslationThetaOffset=0  TranslationThetaOffsetUnits=deg  RotationMethod=None  RotationAngleUnits=deg  RotationStandardAxis=+Z  RotationAngle=0.0  RotationArbitraryAxis=[0 0 1]  FollAlignAxisA=+X  BaseAlignAxisA=+Y  FollAlignAxisB=+Y  BaseAlignAxisB=+Z  RotationSequenceAxes=FollowerAxes  RotationSequence=XYX  RotationSequenceAngles=[0 0 0]  RotationSequenceAnglesUnits=deg  RotationMatrix=[1 0 0; 0 1 0; 0 0 1]
  To Toe-top : sm_lib/Frames and Transforms/Rigid Transform  TranslationMethod=Cartesian  TranslationStandardOffset=0  TranslationLengthUnit=m  TranslationStandardAxis=+Z  TranslationCartesianOffset=[0 ankle_height 0]  TranslationROffset=0  TranslationROffsetUnits=m  TranslationZOffset=0  TranslationZOffsetUnits=m  TranslationThetaOffset=0  TranslationThetaOffsetUnits=deg  RotationMethod=None  RotationAngleUnits=deg  RotationStandardAxis=+Z  RotationAngle=0.0  RotationArbitraryAxis=[0 0 1]  FollAlignAxisA=+X  BaseAlignAxisA=+Y  FollAlignAxisB=+Y  BaseAlignAxisB=+Z  RotationSequenceAxes=FollowerAxes  RotationSequence=XYX  RotationSequenceAngles=[0 0 0]  RotationSequenceAnglesUnits=deg  RotationMatrix=[1 0 0; 0 1 0; 0 0 1]
  To center : sm_lib/Frames and Transforms/Rigid Transform  TranslationMethod=Cartesian  TranslationStandardOffset=0  TranslationLengthUnit=m  TranslationStandardAxis=+Z  TranslationCartesianOffset=[-footLength/2 ankle_height/2 0]  TranslationROffset=0  TranslationROffsetUnits=m  TranslationZOffset=0  TranslationZOffsetUnits=m  TranslationThetaOffset=0  TranslationThetaOffsetUnits=deg  RotationMethod=None  RotationAngleUnits=deg  RotationStandardAxis=+Z  RotationAngle=0.0  RotationArbitraryAxis=[0 0 1]  FollAlignAxisA=+X  BaseAlignAxisA=+Y  FollAlignAxisB=+Y  BaseAlignAxisB=+Z  RotationSequenceAxes=FollowerAxes  RotationSequence=XYX  RotationSequenceAngles=[0 0 0]  RotationSequenceAnglesUnits=deg  RotationMatrix=[1 0 0; 0 1 0; 0 0 1]
  ankle : PMIOPort  Side=Left
  World : PMIOPort  Port=2  Side=Right
  CG : PMIOPort  Port=3  Side=Left
  Ball+ : PMIOPort  Port=4  Side=Right
  Ball- : PMIOPort  Port=5  Side=Right
  Heel+ : PMIOPort  Port=6  Side=Right
  Heel- : PMIOPort  Port=7  Side=Right
  Ball+ top : PMIOPort  Port=8  Side=Right
  Ball- top : PMIOPort  Port=9  Side=Right
  Stance? : Outport  VectorParamsAs1DForOutWhenUnconnected=on
  GRF : Outport  Port=2  VectorParamsAs1DForOutWhenUnconnected=on
  Toe pos : Outport  Port=3  VectorParamsAs1DForOutWhenUnconnected=on
  Heel pos : Outport  Port=4  VectorParamsAs1DForOutWhenUnconnected=on
  wires:
  OR/1 -> Cast To Double1/1
  Ground Contact Model 3D2/1 -> OR/2
  Ground Contact Model 3D2/2 -> Add/2
  Ground Contact Model 3D3/2 -> Add/1
  Ground Contact Model 3D3/1 -> OR/1
  Ground Contact Model 3D/2 -> Add/4
  Ground Contact Model 3D/1 -> OR/4
  Ground Contact Model 3D1/1 -> OR/3
  Add/1 -> Demux/1
  Position Sensor/1 -> Add1/2, Env Lookup/1
  Env Lookup2/1 -> Ground Contact Model 3D3/1
  Position Sensor3/1 -> Add1/1, Env Lookup2/1
  Position Sensor1/1 -> Add2/1, Env Lookup1/1
  Env Lookup3/1 -> Ground Contact Model 3D/1
  Position Sensor2/1 -> Add2/2, Env Lookup3/1
  Cast To Double1/1 -> Stance?/1
  Env Lookup/1 -> Ground Contact Model 3D2/1
  Env Lookup1/1 -> Ground Contact Model 3D1/1
  Ground Contact Model 3D1/2 -> Add/3
  Add1/1 -> Multiply/1
  Multiply/1 -> Toe pos/1
  Multiply1/1 -> Heel pos/1
  Add2/1 -> Multiply1/1
  yaw/1 -> Cos/1, Sin/1
  Cos/1 -> [yawCos]
  Sin/1 -> [yawSin]
  Mux/1 -> GRF/1
  [yawCos] -> Product/1
  Demux/1 -> Product3/1, Product/2  "x_global"
  [yawSin] -> Product1/1
  Demux/2 -> Product1/2, Product2/1  "y_global"
  Add3/1 -> Mux/1  "x_anterior"
  Product1/1 -> Add3/2
  Product/1 -> Add3/1
  Add4/1 -> Product4/1
  [yawCos] -> Product2/2
  [yawSin] -> Product3/2
  Product2/1 -> Add4/2
  Product3/1 -> Add4/1
  Demux/3 -> Mux/3  "z"
  Product4/1 -> Mux/2  "y_mediolateral"
  Compare To Constant1/1 -> Cast To Double2/1  "rightside"
  Compare To Constant/1 -> Cast To Double/1  "leftside"
  Constant/1 -> Compare To Constant1/1, Compare To Constant/1
  Add5/1 -> Product4/2
  Cast To Double/1 -> Add5/1  "leftside"
  Cast To Double2/1 -> Add5/2  "rightside"
  connections:
  Ground Contact Model 3D/LConn1 -- Position Sensor2/LConn1 -- Heel-/RConn1 -- To Heel-/RConn1
  Position Sensor1/LConn1 -- To Heel+/RConn1 -- Ground Contact Model 3D1/LConn1 -- Heel+/RConn1
  Position Sensor3/LConn1 -- To Toe-top/LConn1 -- To Ball+/RConn1 -- Ground Contact Model 3D3/LConn1 -- Ball+/RConn1
  To Ball-/RConn1 -- Rigid Transform/LConn1 -- Position Sensor/LConn1 -- Ground Contact Model 3D2/LConn1 -- Ball-/RConn1
  To CG/RConn1 -- Inertia/RConn1 -- CG/RConn1
  To CG/LConn1 -- World/RConn1 -- To center/LConn1 -- To Ball+/LConn1 -- To Ball-/LConn1 -- To Heel-/LConn1 -- To Heel+/LConn1 -- Foot to Ankle/LConn1
  Brick Solid/RConn1 -- To center/RConn1
  Foot to Ankle/RConn1 -- ankle/RConn1
  To Toe-top/RConn1 -- Ball+ top/RConn1
  Ball- top/RConn1 -- Rigid Transform/RConn1

== system NeuroMuscularLibrary/Force Plate ==
  "GRF_Ball [N N] " : Inport
  GRF_Heel [N N] : Inport  Port=2
  Enable : EnablePort  StatesWhenEnabling=reset
  Fcn : Fcn  Expr=u(1)/(u(2)+eps)
  Mux : Mux  Inputs=3
  Mux1 : Mux  Inputs=2
  Selector : Selector  InputPortWidth=2  IndexOptions=Index vector (dialog)  Indices=2  OutputSizes=1
  Selector1 : Selector  InputPortWidth=2  IndexOptions=Index vector (dialog)  Indices=2  OutputSizes=1
  Sum1 : Sum
  GRFs : Outport  OutputWhenDisabled=reset  InitialOutput=0  VectorParamsAs1DForOutWhenUnconnected=on
  COP : Outport  Port=2  OutputWhenDisabled=reset  InitialOutput=0  VectorParamsAs1DForOutWhenUnconnected=on
  wires:
  Selector/1 -> Mux1/2
  Selector1/1 -> Mux1/1
  "GRF_Ball [N N] "/1 -> Sum1/1, Mux/1, Selector1/1
  GRF_Heel [N N]/1 -> Sum1/2, Mux/3
  Sum1/1 -> Mux/2, Selector/1
  Mux/1 -> GRFs/1
  Mux1/1 -> Fcn/1
  Fcn/1 -> COP/1

== system NeuroMuscularLibrary/GAS Link ==
  note: GAS Attachment
  Knee angle [rad] : Inport
  Ankle angle [rad] : Inport  Port=2
  Constant1 : Constant  Value=phimaxGASk
  Constant2 : Constant  Value=phirefGASk
  Constant3 : Constant  Value=phimaxGASa
  Constant4 : Constant  Value=lslackGAS+loptGAS
  Constant5 : Constant  Value=phirefGASa
  Demux : Demux  Outputs=2
  Demux1 : Demux  Outputs=2
  Gain1 : Gain  Gain=rGASkmax
  Gain2 : Gain  Gain=rGASamax
  Gain3 : Gain  Gain=phiScaleGASa
  Gain5 : Gain  Gain=phiScaleGASk
  Gain6 : Gain  Gain=phiScaleGASk
  Gain7 : Gain  Gain=rhoGASk/phiScaleGASk
  Gain8 : Gain  Gain=phiScaleGASa
  Gain9 : Gain  Gain=rhoGASa/phiScaleGASa
  Mux : Mux  Inputs=2
  Mux1 : Mux  Inputs=2
  Sum1 : Sum  Inputs=-+
  Sum2 : Sum  Inputs=|+-
  Sum3 : Sum  Inputs=-+|
  Sum4 : Sum  Inputs=-+
  Sum5 : Sum  Inputs=-+-
  Sum6 : Sum  Inputs=|+-
  Sum7 : Sum  Inputs=-+|
  length change term : Trigonometry
  length change term1 : Trigonometry
  offset correction term : Trigonometry
  offset correction term1 : Trigonometry
  variable lever term : Trigonometry  Operator=cos
  variable lever term1 : Trigonometry  Operator=cos
  lmtu [m] : Outport  VectorParamsAs1DForOutWhenUnconnected=on
  leverKnee [m] : Outport  Port=2  VectorParamsAs1DForOutWhenUnconnected=on
  leverAnkle [m] : Outport  Port=3  VectorParamsAs1DForOutWhenUnconnected=on
  wires:
  Sum4/1 -> Mux1/1
  Gain8/1 -> offset correction term1/1
  Gain7/1 -> Sum5/1
  Demux1/2 -> leverAnkle [m]/1
  Constant4/1 -> Sum5/2
  Sum5/1 -> lmtu [m]/1
  Demux1/1 -> Gain9/1
  Mux1/1 -> Gain2/1
  Sum2/1 -> Gain6/1
  Gain2/1 -> Demux1/1
  offset correction term1/1 -> Sum4/1
  Gain6/1 -> offset correction term/1
  length change term1/1 -> Sum4/2
  variable lever term/1 -> Mux/2
  Constant5/1 -> Sum6/1
  Demux/2 -> leverKnee [m]/1
  Sum6/1 -> Gain8/1
  Gain1/1 -> Demux/1
  Mux/1 -> Gain1/1
  Sum1/1 -> Mux/1
  Constant3/1 -> Sum7/1, Sum6/2
  Sum7/1 -> Gain3/1
  Gain5/1 -> variable lever term/1, length change term/1
  offset correction term/1 -> Sum1/1
  variable lever term1/1 -> Mux1/2
  Constant1/1 -> Sum3/1, Sum2/2
  Gain9/1 -> Sum5/3
  Constant2/1 -> Sum2/1
  length change term/1 -> Sum1/2
  Gain3/1 -> variable lever term1/1, length change term1/1
  Sum3/1 -> Gain5/1
  Knee angle [rad]/1 -> Sum3/2
  Ankle angle [rad]/1 -> Sum7/2
  Demux/1 -> Gain7/1

== system NeuroMuscularLibrary/GLU Link ==
  note: GLUTEUS Attachment
  hip angle [rad] : Inport
  Constant : Constant  Value=lslackGLU+loptGLU
  Constant1 : Constant  Value=rGLU
  Constant2 : Constant  Value=phirefGLU
  Gain2 : Gain  Gain=rhoGLU
  Product : Product  RndMeth=Zero
  Sum2 : Sum  Inputs=|+-
  Sum5 : Sum  Inputs=|+-
  lmtu [m] : Outport  VectorParamsAs1DForOutWhenUnconnected=on
  lever [m] : Outport  Port=2  VectorParamsAs1DForOutWhenUnconnected=on
  wires:
  Constant/1 -> Sum5/1
  Sum5/1 -> lmtu [m]/1
  Product/1 -> Gain2/1
  Constant2/1 -> Sum2/2
  Sum2/1 -> Product/1
  Constant1/1 -> Product/2, lever [m]/1
  Gain2/1 -> Sum5/2
  hip angle [rad]/1 -> Sum2/1

== system NeuroMuscularLibrary/Global2LocalAxes ==
  note: Left hip(+)/Right hip(-)
  note: Front(+)/Back(-)
  note: Up(+)/Down(-)
  "Global " : Inport
  yaw : Inport  Port=2
  Add3 : Sum
  Add4 : Sum  Inputs=-+
  Cos : Trigonometry  Operator=cos
  Demux : Demux  Outputs=3
  Mux : Mux  Inputs=3
  Product{,1..3} (4 alike) : Product
  Sin : Trigonometry
  Local : Outport  VectorParamsAs1DForOutWhenUnconnected=on
  wires:
  Demux/1 -> Product3/1, Product/2  "x_global"
  [yawSin] -> Product1/1
  [yawCos] -> Product/1
  Demux/3 -> Mux/3  "z"
  Add4/1 -> Mux/2  "y_local"
  Product3/1 -> Add4/1
  "Global "/1 -> Demux/1
  Demux/2 -> Product1/2, Product2/1  "y_global"
  Mux/1 -> Local/1
  Product2/1 -> Add4/2
  Product/1 -> Add3/1
  Add3/1 -> Mux/1  "x_local"
  [yawCos] -> Product2/2
  [yawSin] -> Product3/2
  Product1/1 -> Add3/2
  yaw/1 -> Cos/1, Sin/1
  Cos/1 -> [yawCos]
  Sin/1 -> [yawSin]
